simulink model "mod_assign"  (R2019b)
settings: Solver=VariableStepAuto  StartTime=0.0  StopTime=10.0  RelTol=1e-3
undefined symbols (not defined in the file or in its folder): angularMon, damp, ki, kp, powerNew, powerSet, rGovern, timeChanging
settings Model: Creator=edxu96  LastModifiedBy=edxu96

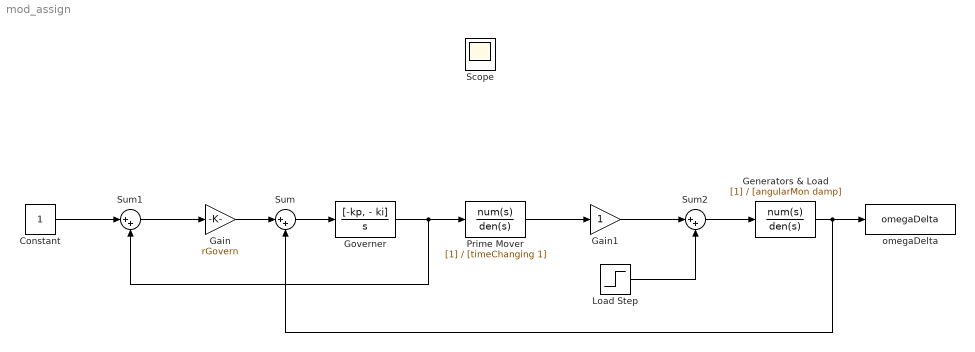
== system mod_assign ==
  Constant : Constant
  Gain : Gain  Gain=rGovern
  Gain1 : Gain
  Generators & Load : TransferFcn  Denominator=[angularMon damp]
  Governer : TransferFcn  Numerator=[-kp, - ki]  Denominator=[1, 0]
  Load Step : Step  Time=0  Before=powerSet  After=powerNew  SampleTime=0
  Prime Mover : TransferFcn  Denominator=[timeChanging 1]
  Scope : Scope
  Sum : Sum  Inputs=|++
  Sum1 : Sum  Inputs=|++
  Sum2 : Sum  Inputs=|++
  omegaDelta : ToWorkspace  VariableName=omegaDelta  SaveFormat=Timeseries  SampleTime=-1
  wires:
  Gain/1 -> Sum/1
  Constant/1 -> Sum1/1
  Sum1/1 -> Gain/1
  Sum/1 -> Governer/1
  Governer/1 -> Sum1/2, Prime Mover/1
  Prime Mover/1 -> Gain1/1
  Gain1/1 -> Sum2/1
  Sum2/1 -> Generators & Load/1
  Generators & Load/1 -> Sum/2, omegaDelta/1
  Load Step/1 -> Sum2/2
